simulink model "calcAeroLoadsInBdyFrame_th"  (R2020a)
settings: Solver=VariableStepAuto  StartTime=0.0  StopTime=4  MaxStep=0.05  RelTol=1e-3
libraries: calcAeroLoadsInBdyFrame_cl x1
settings Model: Creator=Ayaz  LastModifiedBy=Ayaz

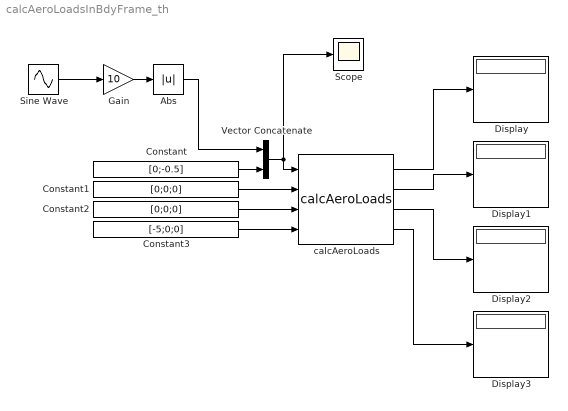
== system calcAeroLoadsInBdyFrame_th ==
  Abs : Abs
  Constant : Constant  Value=[0;-0.5]  VectorParams1D=off
  Constant1 : Constant  Value=[0;0;0]  VectorParams1D=off
  Constant2 : Constant  Value=[0;0;0]  VectorParams1D=off
  Constant3 : Constant  Value=[-5;0;0]  VectorParams1D=off
  Display{,1..3} (4 alike) : Display
  Gain : Gain  Gain=10
  Scope : Scope
  Sine Wave : Sin  Frequency=0.25*2*pi  SampleTime=0
  Vector Concatenate : Concatenate
  calcAeroLoads : calcAeroLoadsInBdyFrame_cl/calcAeroLoads  refArea=3  refSpan=5.5  refChord=0.55  rho=1.225
  wires:
  Constant/1 -> Vector Concatenate/2
  Constant1/1 -> calcAeroLoads/2
  Constant2/1 -> calcAeroLoads/3
  Constant3/1 -> calcAeroLoads/4
  calcAeroLoads/2 -> Display1/1
  calcAeroLoads/1 -> Display/1
  Sine Wave/1 -> Gain/1
  Vector Concatenate/1 -> Scope/1, calcAeroLoads/1
  Gain/1 -> Abs/1
  Abs/1 -> Vector Concatenate/1
  calcAeroLoads/3 -> Display2/1
  calcAeroLoads/4 -> Display3/1
